simulink model "FC_Test"  (R2023b)
settings: Solver=FixedStepAuto  StartTime=0.0  StopTime=inf  RelTol=1e-3  EnableMultiTasking=on
PreLoadFcn:
  | setupEnv()
undefined symbols (not defined in the file or in its folder): bits, sensors
libraries: stm32blockslib x31, simulink x7, stm32f4xxblockslib x2
settings Model: STM32="{\"DigitalPortRead\":{\"ID\":\"FC_Test:2\"},\"DigitalPortWrite\":{\"ID\":\"FC_Test:4\"},\"I2CControllerRead\":[{\"ID\":\"FC_Test:28\"},{\"ID\":\"FC_Test:50\"},{\"ID\":\"FC_Test:52\"},{\"ID\":\"FC_Test:53\"},{\"ID\":\"FC_Test:68\"},{\"ID\":\"FC_Test:96\"},{\"ID\":\"FC_Test:191\"},{\"ID\":\"FC_Test:128\"},{\"ID\":\"FC_Test:121\"},{\"ID\":\"FC_Test:169\"},{\"ID\":\"FC_Test:249\"},{\"ID\":\"FC_Test:250\"},{\"ID\":\"FC_Test:237\"}],\"I2CControllerWrite\":[{\"ID\":\"FC_Test:86\"},{\"ID\":\"FC_Test:109\"},{\"ID\":\"FC_Test:94\"},{\"ID\":\"FC_Test:208\"},{\"ID\":\"FC_Test:192\"},{\"ID\":\"FC_Test:202\"},{\"ID\":\"FC_Test:140\"},{\"ID\":\"FC_Test:141\"},{\"ID\":\"FC_Test:142\"},{\"ID\":\"FC_Test:122\"},{\"ID\":\"FC_Test:170\"},{\"ID\":\"FC_Test:239\"},{\"ID\":\"FC_Test:242\"},{\"ID\":\"FC_Test:243\"},{\"ID\":\"FC_Test:246\"},{\"ID\":\"FC_Test:247\"},{\"ID\":\"FC_Test:255\"},{\"ID\":\"FC_Test:252\"}]}"  SimulationMode=external  Creator=Blind  LastModifiedBy=Blind
settings SolverCC: PositivePriorityOrder=on
settings OptimizationCC: EnhancedBackFolding=on  PassReuseOutputArgsAs=Individual arguments  ZeroExternalMemoryAtStartup=off  ZeroInternalMemoryAtStartup=off  MaxStackSize=64  OptimizeBlockOrder=speed  DifferentSizesBufferReuse=on  OptimizationCustomize=off  EfficientTunableParamExpr=on
settings DebuggingCC: ParameterTunabilityLossMsg=error
settings HardwareCC: ProdBitPerPointer=32  ProdBitPerSizeT=32  ProdBitPerPtrDiffT=32  ProdLargestAtomicInteger=Long  ProdLargestAtomicFloat=Double  ProdWordSize=32  ProdLongLongMode=on  ProdHWDeviceType=ARM Compatible->ARM Cortex
settings SFSimCC: MATLABDynamicMemAlloc=off
settings RTWCC: Description=Embedded Coder  SystemTargetFile=ert.tlc  HardwareBoard=STM32H7xx Based (Single-core)  TLCOptions="-aInlineSetEventsForThisBaseRateFcn=TLC_FALSE -aSuppressMultiTaskScheduler=TLC_FALSE   -aRateBasedStepFcn=1"  TemplateMakefile=ert_default_tmf  Toolchain=GNU Tools for ARM Embedded Processors
settings CodeAppCC: ForceParamTrailComments=on  IgnoreCustomStorageClasses=off  OperatorAnnotations=on  SimulinkDataObjDesc=on  SFDataObjDesc=on  InsertBlockDesc=on
settings ERTTargetCC: CodeReplacementLibrary=ARM Cortex-M  SupportContinuousTime=on  ExtModeTransport=3  ExtModeStaticAlloc=on  ExtModeStaticAllocSize=4096  ExtModeMexFile=ext_xcp  ExtModeIntrfLevel=Level2 - Open

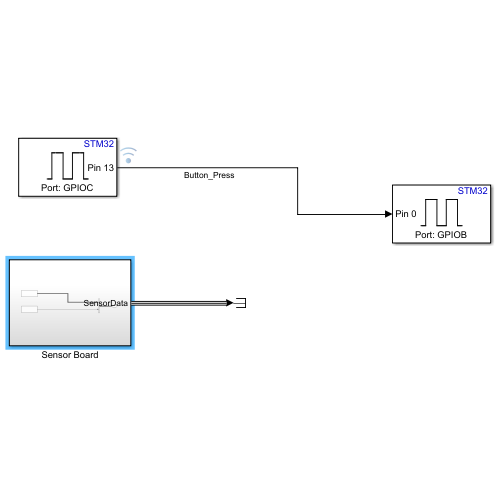
[thumbnail: Simulink's stored preview of the top-level diagram]
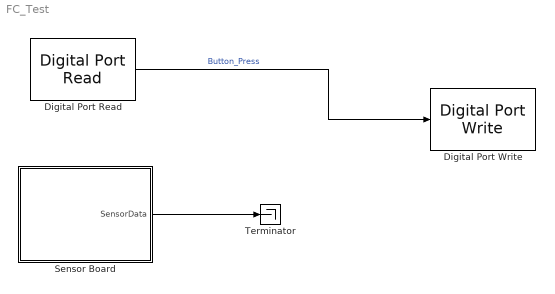
== system FC_Test ==
  Digital Port Read : stm32f4xxblockslib/Digital Port Read  PortName=GPIOC  PinNumber=13  ReadOperation=on  IOAsArray=off  SampleTime=-1  EnableSimPort=off  hoistedMaskSrc=ECSoC/ECSimCodegen/Digital Port Read
      settings: LibrarySourceBlock=stm32h7xxblockslib/Digital Port Read
  Digital Port Write : stm32f4xxblockslib/Digital Port Write  PortName=GPIOB  PinNumber=0  ReadOperation=off  IOAsArray=off  EnableSimPort=off  hoistedMaskSrc=ECSoC/ECSimCodegen/Digital Port Write
      settings: LibrarySourceBlock=stm32h7xxblockslib/Digital Port Write
  Sensor Board : Subsystem
  Terminator : Terminator
  wires:
  Digital Port Read/1 -> Digital Port Write/1  "Button_Press"
  Sensor Board/1(SensorData) -> Terminator/1

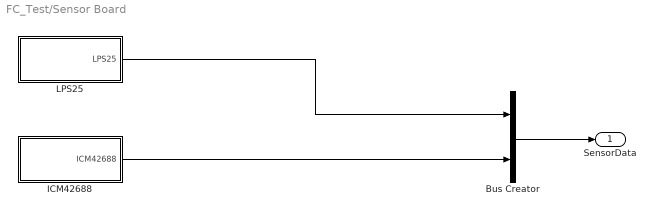
== system FC_Test/Sensor Board ==
  Bus Creator : BusCreator  Inputs=2
  ICM42688 : Subsystem
  LPS25 : Subsystem
  SensorData : Outport
  wires:
  LPS25/1(LPS25) -> Bus Creator/1
  Bus Creator/1 -> SensorData/1
  ICM42688/1(ICM42688) -> Bus Creator/2

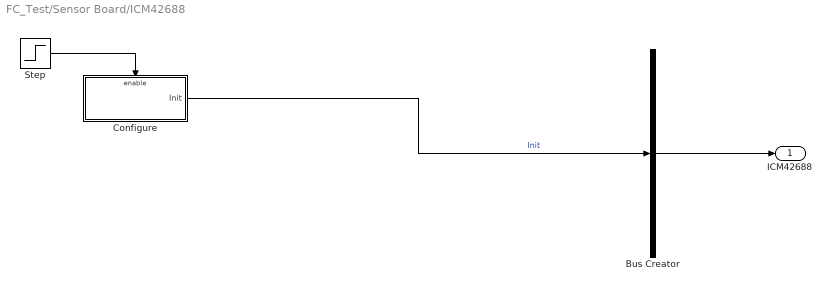
== system FC_Test/Sensor Board/ICM42688 ==
  Bus Creator : BusCreator  Inputs=1
  Configure : Subsystem
  Step : Step  Time=0  SampleTime=0
  ICM42688 : Outport
  wires:
  Configure/1(Init) -> Bus Creator/1  "Init"
  Step/1 -> Configure/Enable
  Bus Creator/1 -> ICM42688/1

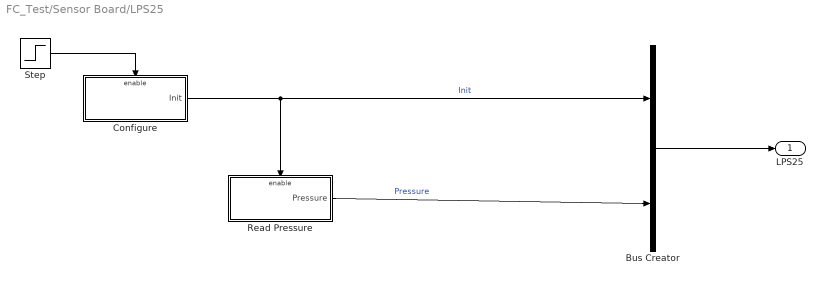
== system FC_Test/Sensor Board/LPS25 ==
  Bus Creator : BusCreator  Inputs=2
  Configure : Subsystem
  Read Pressure : Subsystem
  Step : Step  Time=0  SampleTime=0
  LPS25 : Outport
  wires:
  Step/1 -> Configure/Enable
  Read Pressure/1(Pressure) -> Bus Creator/2  "Pressure"
  Bus Creator/1 -> LPS25/1
  Configure/1(Init) -> Bus Creator/1, Read Pressure/Enable  "Init"

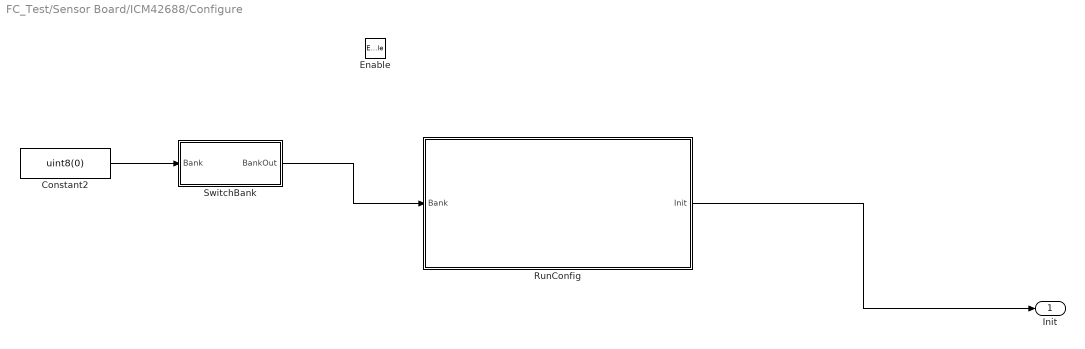
== system FC_Test/Sensor Board/ICM42688/Configure ==
  Enable : EnablePort
  Constant2 : Constant  Value=uint8(0)
  RunConfig : Subsystem
  SwitchBank : Subsystem
  Init : Outport
  wires:
  Constant2/1 -> SwitchBank/1(Bank)
  RunConfig/1(Init) -> Init/1
  SwitchBank/1(BankOut) -> RunConfig/1(Bank)

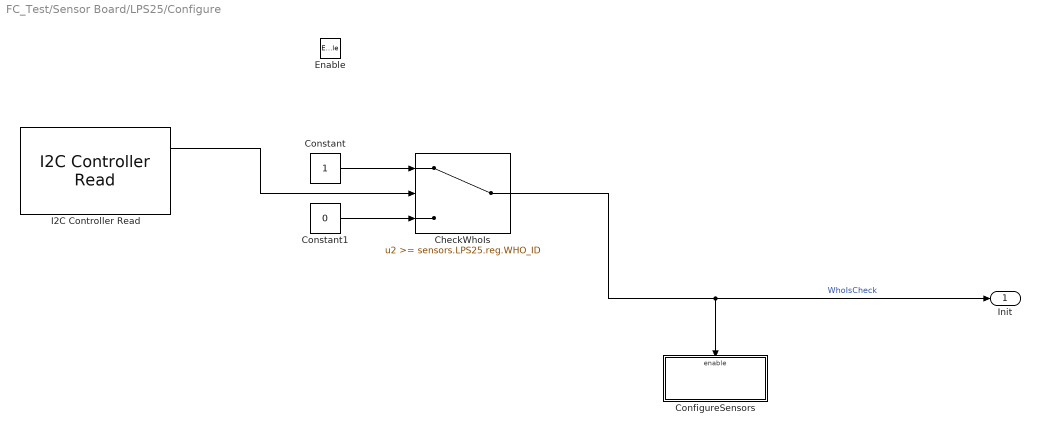
== system FC_Test/Sensor Board/LPS25/Configure ==
  Enable : EnablePort
  CheckWhoIs : Switch  Threshold=sensors.LPS25.reg.WHO_ID  SaturateOnIntegerOverflow=off  InputSameDT=off
  ConfigureSensors : Subsystem
  Constant : Constant
  Constant1 : Constant  Value=0
  I2C Controller Read : stm32blockslib/I2C Controller Read  I2CModule=I2C1  Mode=Controller  AddressingMode=7-bits  PeripheralByteOrder=BigEndian  OwnPeripheralAddress=uint8(170)  PeripheralAddressVia=Dialog  PeripheralAddress=sensors.LPS25.reg.ADDR  RegisterAddressMode=on  RegisterAddressVia=Dialog  RegisterAddress=sensors.LPS25.reg.WHOAMI  RepeatedStart=off  NoAck=off  OutputStatus=on  BlockMode=Receive  DataType=uint8  DataLength=1  Timeout=0.001  SampleTime=-1
      settings: LibrarySourceBlock=stm32h7xxblockslib/I2C Controller Read
  Init : Outport
  wires:
  I2C Controller Read/1 -> CheckWhoIs/2
  Constant/1 -> CheckWhoIs/1
  Constant1/1 -> CheckWhoIs/3
  CheckWhoIs/1 -> ConfigureSensors/Enable, Init/1  "WhoIsCheck"

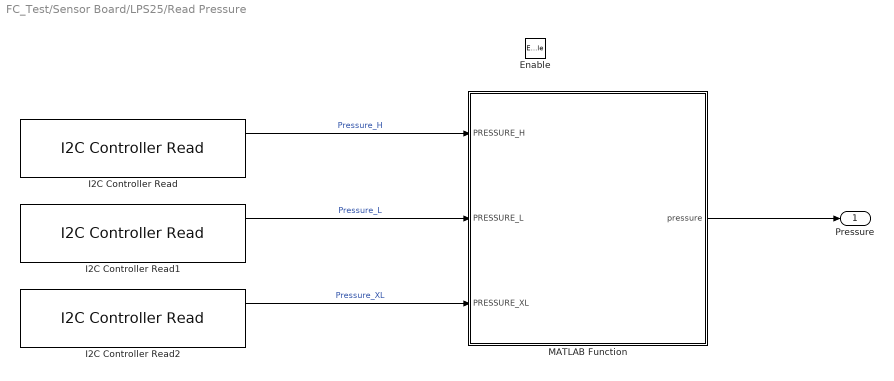
== system FC_Test/Sensor Board/LPS25/Read Pressure ==
  Enable : EnablePort
  I2C Controller Read : stm32blockslib/I2C Controller Read  I2CModule=I2C1  Mode=Controller  AddressingMode=7-bits  PeripheralByteOrder=BigEndian  OwnPeripheralAddress=uint8(170)  PeripheralAddressVia=Dialog  PeripheralAddress=sensors.LPS25.reg.ADDR  RegisterAddressMode=on  RegisterAddressVia=Dialog  RegisterAddress=sensors.LPS25.reg.PRESSURE_H_REG  RepeatedStart=off  NoAck=off  OutputStatus=on  BlockMode=Receive  DataType=uint8  DataLength=1  Timeout=0.001  SampleTime=-1
      settings: LibrarySourceBlock=stm32h7xxblockslib/I2C Controller Read
  I2C Controller Read1 : stm32blockslib/I2C Controller Read  I2CModule=I2C1  Mode=Controller  AddressingMode=7-bits  PeripheralByteOrder=BigEndian  OwnPeripheralAddress=uint8(170)  PeripheralAddressVia=Dialog  PeripheralAddress=sensors.LPS25.reg.ADDR  RegisterAddressMode=on  RegisterAddressVia=Dialog  RegisterAddress=sensors.LPS25.reg.PRESSURE_L_REG  RepeatedStart=off  NoAck=off  OutputStatus=on  BlockMode=Receive  DataType=uint8  DataLength=1  Timeout=0.001  SampleTime=-1
      settings: LibrarySourceBlock=stm32h7xxblockslib/I2C Controller Read
  I2C Controller Read2 : stm32blockslib/I2C Controller Read  I2CModule=I2C1  Mode=Controller  AddressingMode=7-bits  PeripheralByteOrder=BigEndian  OwnPeripheralAddress=uint8(170)  PeripheralAddressVia=Dialog  PeripheralAddress=sensors.LPS25.reg.ADDR  RegisterAddressMode=on  RegisterAddressVia=Dialog  RegisterAddress=sensors.LPS25.reg.PRESSURE_OUT_XL  RepeatedStart=off  NoAck=off  OutputStatus=on  BlockMode=Receive  DataType=uint8  DataLength=1  Timeout=0.001  SampleTime=-1
      settings: LibrarySourceBlock=stm32h7xxblockslib/I2C Controller Read
  MATLAB Function : MATLAB Function  TreatAsAtomicUnit=on
  Pressure : Outport
  wires:
  I2C Controller Read/1 -> MATLAB Function/1(PRESSURE_H)  "Pressure_H"
  I2C Controller Read1/1 -> MATLAB Function/2(PRESSURE_L)  "Pressure_L"
  I2C Controller Read2/1 -> MATLAB Function/3(PRESSURE_XL)  "Pressure_XL"
  MATLAB Function/1(pressure) -> Pressure/1

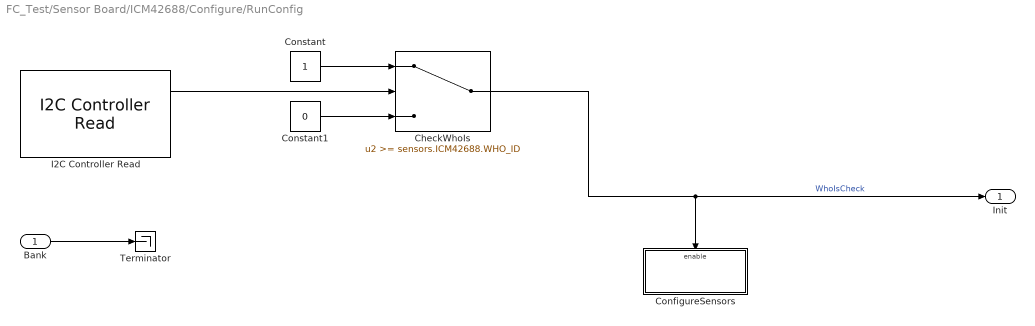
== system FC_Test/Sensor Board/ICM42688/Configure/RunConfig ==
  Bank : Inport
  CheckWhoIs : Switch  Threshold=sensors.ICM42688.WHO_ID  SaturateOnIntegerOverflow=off  InputSameDT=off
  ConfigureSensors : Subsystem
  Constant : Constant
  Constant1 : Constant  Value=0
  I2C Controller Read : stm32blockslib/I2C Controller Read  I2CModule=I2C1  Mode=Controller  AddressingMode=7-bits  PeripheralByteOrder=BigEndian  OwnPeripheralAddress=uint8(170)  PeripheralAddressVia=Dialog  PeripheralAddress=sensors.ICM42688.reg.ADDR  RegisterAddressMode=on  RegisterAddressVia=Dialog  RegisterAddress=sensors.ICM42688.reg.BANK0.WHO_AM_I  RepeatedStart=off  NoAck=off  OutputStatus=on  BlockMode=Receive  DataType=uint8  DataLength=1  Timeout=0.001  SampleTime=-1
      settings: LibrarySourceBlock=stm32h7xxblockslib/I2C Controller Read
  Terminator : Terminator
  Init : Outport
  wires:
  I2C Controller Read/1 -> CheckWhoIs/2
  CheckWhoIs/1 -> Init/1, ConfigureSensors/Enable  "WhoIsCheck"
  Constant/1 -> CheckWhoIs/1
  Constant1/1 -> CheckWhoIs/3
  Bank/1 -> Terminator/1

== system FC_Test/Sensor Board/ICM42688/Configure/SwitchBank ==
  Bank : Inport
  I2C Controller Read : stm32blockslib/I2C Controller Read  I2CModule=I2C1  Mode=Controller  AddressingMode=7-bits  PeripheralByteOrder=BigEndian  OwnPeripheralAddress=uint8(170)  PeripheralAddressVia=Dialog  PeripheralAddress=sensors.ICM42688.reg.ADDR  RegisterAddressMode=on  RegisterAddressVia=Dialog  RegisterAddress=sensors.ICM42688.reg.REG_BANK_SEL  RepeatedStart=off  NoAck=off  OutputStatus=on  BlockMode=Receive  DataType=uint8  DataLength=1  Timeout=0.001  SampleTime=-1
      settings: LibrarySourceBlock=stm32h7xxblockslib/I2C Controller Read
  I2C Controller Write : stm32blockslib/I2C Controller Write  I2CModule=I2C1  Mode=Controller  AddressingMode=7-bits  PeripheralByteOrder=BigEndian  OwnPeripheralAddress=uint8(170)  PeripheralAddressVia=Dialog  PeripheralAddress=sensors.ICM42688.reg.ADDR  RegisterAddressMode=on  RegisterAddressVia=Dialog  RegisterAddress=sensors.ICM42688.reg.REG_BANK_SEL  RepeatedStart=off  NoAck=off  OutputStatus=on  BlockMode=Transmit  DataType=uint8  DataLength=1  Timeout=0.001  SampleTime=-1
      settings: LibrarySourceBlock=stm32h7xxblockslib/I2C Controller Write
  BankOut : Outport
  wires:
  Bank/1 -> I2C Controller Write/1
  I2C Controller Read/1 -> BankOut/1

== system FC_Test/Sensor Board/LPS25/Configure/ConfigureSensors ==
  Enable : EnablePort
  Constant : Constant  Value=sensors.LPS25.config.ODR.Hz25
  I2C Controller Write : stm32blockslib/I2C Controller Write  I2CModule=I2C1  Mode=Controller  AddressingMode=7-bits  PeripheralByteOrder=BigEndian  OwnPeripheralAddress=uint8(170)  PeripheralAddressVia=Dialog  PeripheralAddress=sensors.LPS25.reg.ADDR  RegisterAddressMode=on  RegisterAddressVia=Dialog  RegisterAddress=sensors.LPS25.reg.CTRL1  RepeatedStart=off  NoAck=off  OutputStatus=on  BlockMode=Transmit  DataType=uint8  DataLength=1  Timeout=0.001  SampleTime=-1
      settings: LibrarySourceBlock=stm32h7xxblockslib/I2C Controller Write
  wires:
  Constant/1 -> I2C Controller Write/1

== system FC_Test/Sensor Board/ICM42688/Configure/RunConfig/ConfigureSensors ==
  Enable : EnablePort
  EnableSensor : Subsystem
  SetFilters : Subsystem
  SetODR : Subsystem

== system FC_Test/Sensor Board/ICM42688/Configure/RunConfig/ConfigureSensors/EnableSensor ==
  Constant : Constant  Value=sensors.ICM42688.config.SENSOR_ENABLE
  I2C Controller Write : stm32blockslib/I2C Controller Write  I2CModule=I2C1  Mode=Controller  AddressingMode=7-bits  PeripheralByteOrder=BigEndian  OwnPeripheralAddress=uint8(170)  PeripheralAddressVia=Dialog  PeripheralAddress=sensors.ICM42688.reg.ADDR  RegisterAddressMode=on  RegisterAddressVia=Dialog  RegisterAddress=sensors.ICM42688.reg.BANK0.PWR_MGMT0  RepeatedStart=off  NoAck=off  OutputStatus=on  BlockMode=Transmit  DataType=uint8  DataLength=1  Timeout=0.001  SampleTime=-1
      settings: LibrarySourceBlock=stm32h7xxblockslib/I2C Controller Write
  Status : Outport
  wires:
  Constant/1 -> I2C Controller Write/1
  I2C Controller Write/1 -> Status/1

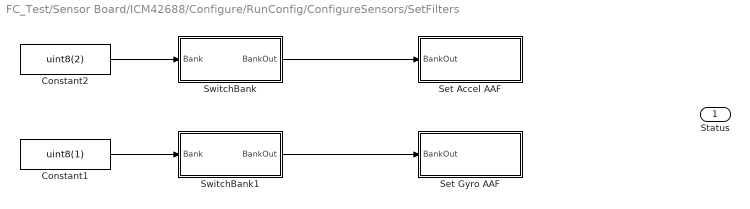
== system FC_Test/Sensor Board/ICM42688/Configure/RunConfig/ConfigureSensors/SetFilters ==
  Constant1 : Constant  Value=uint8(1)
  Constant2 : Constant  Value=uint8(2)
  Set Accel AAF : Subsystem
  Set Gyro AAF : Subsystem
  SwitchBank : Subsystem
  SwitchBank1 : Subsystem
  Status : Outport
  wires:
  Constant2/1 -> SwitchBank/1(Bank)
  SwitchBank/1(BankOut) -> Set Accel AAF/1(BankOut)
  Constant1/1 -> SwitchBank1/1(Bank)
  SwitchBank1/1(BankOut) -> Set Gyro AAF/1(BankOut)

== system FC_Test/Sensor Board/ICM42688/Configure/RunConfig/ConfigureSensors/SetODR ==
  Constant1 : Constant  Value=uint8(0)
  ODR : Subsystem
  SwitchBank1 : Subsystem
  Status : Outport
  wires:
  Constant1/1 -> SwitchBank1/1(Bank)
  SwitchBank1/1(BankOut) -> ODR/1(BankOut)
  ODR/1(Out1) -> Status/1

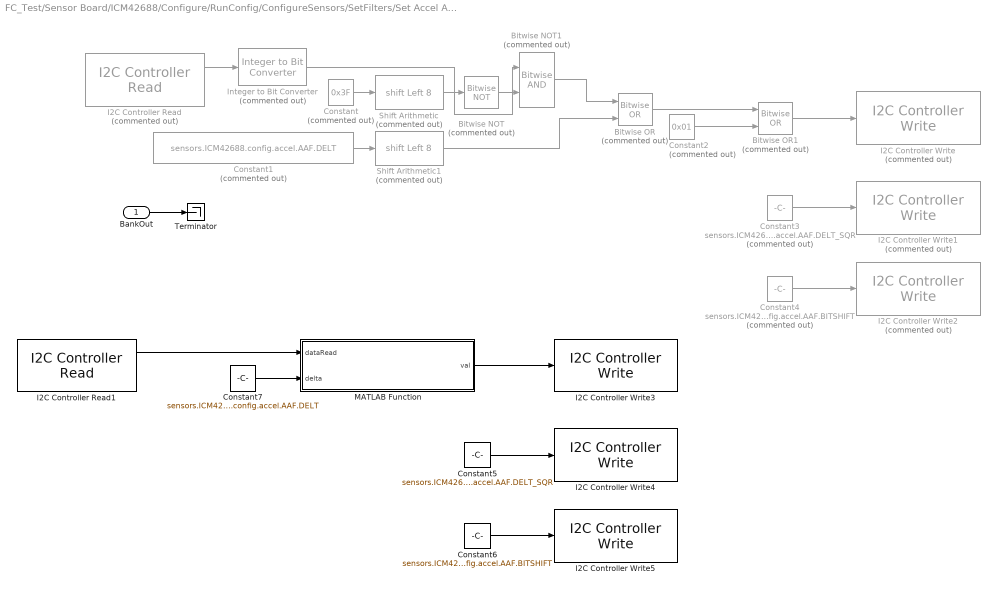
== system FC_Test/Sensor Board/ICM42688/Configure/RunConfig/ConfigureSensors/SetFilters/Set Accel AAF ==
  BankOut : Inport
  Bitwise NOT : simulink/Logic and Bit Operations/Bitwise Operator  Commented=on  logicop=NOT  UseBitMask=off  BitMask=bin2dec('11011001')  BitMaskRealWorld=Stored Integer
      settings: LibrarySourceBlock=|
      | simulink/Quick Insert/Logic and Bit
      | Operations/Bitwise NOT
  Bitwise NOT1 : simulink/Logic and Bit Operations/Bitwise Operator  Commented=on  logicop=AND  UseBitMask=off  NumInputPorts=2  BitMask=bin2dec('11011001')  BitMaskRealWorld=Stored Integer
      settings: LibrarySourceBlock=|
      | simulink/Quick Insert/Logic and Bit
      | Operations/Bitwise NOT
  Bitwise OR : simulink/Logic and Bit Operations/Bitwise Operator  Commented=on  logicop=OR  UseBitMask=off  NumInputPorts=2  BitMask=bin2dec('11011001')  BitMaskRealWorld=Stored Integer
      settings: LibrarySourceBlock=|
      | simulink/Quick Insert/Logic and Bit
      | Operations/Bitwise OR
  Bitwise OR1 : simulink/Logic and Bit Operations/Bitwise Operator  Commented=on  logicop=OR  UseBitMask=off  NumInputPorts=2  BitMask=bin2dec('11011001')  BitMaskRealWorld=Stored Integer
      settings: LibrarySourceBlock=|
      | simulink/Quick Insert/Logic and Bit
      | Operations/Bitwise OR
  Constant : Constant  Commented=on  Value=0x3F
  Constant1 : Constant  Commented=on  Value=sensors.ICM42688.config.accel.AAF.DELT
  Constant2 : Constant  Commented=on  Value=0x01
  Constant3 : Constant  Commented=on  Value=sensors.ICM42688.config.accel.AAF.DELT_SQR
  Constant4 : Constant  Commented=on  Value=sensors.ICM42688.config.accel.AAF.BITSHIFT
  Constant5 : Constant  Value=sensors.ICM42688.config.accel.AAF.DELT_SQR
  Constant6 : Constant  Value=sensors.ICM42688.config.accel.AAF.BITSHIFT
  Constant7 : Constant  Value=sensors.ICM42688.config.accel.AAF.DELT
  I2C Controller Read : stm32blockslib/I2C Controller Read  Commented=on  I2CModule=I2C1  Mode=Controller  AddressingMode=7-bits  PeripheralByteOrder=BigEndian  OwnPeripheralAddress=uint8(170)  PeripheralAddressVia=Dialog  PeripheralAddress=sensors.ICM42688.reg.ADDR  RegisterAddressMode=on  RegisterAddressVia=Dialog  RegisterAddress=sensors.ICM42688.reg.BANK2.ACCEL_CONFIG_STATIC2  RepeatedStart=off  NoAck=off  OutputStatus=on  BlockMode=Receive  DataType=uint8  DataLength=1  Timeout=0.001  SampleTime=-1
      settings: LibrarySourceBlock=stm32h7xxblockslib/I2C Controller Read
  I2C Controller Read1 : stm32blockslib/I2C Controller Read  I2CModule=I2C1  Mode=Controller  AddressingMode=7-bits  PeripheralByteOrder=BigEndian  OwnPeripheralAddress=uint8(170)  PeripheralAddressVia=Dialog  PeripheralAddress=sensors.ICM42688.reg.ADDR  RegisterAddressMode=on  RegisterAddressVia=Dialog  RegisterAddress=sensors.ICM42688.reg.BANK2.ACCEL_CONFIG_STATIC2  RepeatedStart=off  NoAck=off  OutputStatus=on  BlockMode=Receive  DataType=uint8  DataLength=1  Timeout=0.001  SampleTime=-1
      settings: LibrarySourceBlock=stm32h7xxblockslib/I2C Controller Read
  I2C Controller Write : stm32blockslib/I2C Controller Write  Commented=on  I2CModule=I2C1  Mode=Controller  AddressingMode=7-bits  PeripheralByteOrder=BigEndian  OwnPeripheralAddress=uint8(170)  PeripheralAddressVia=Dialog  PeripheralAddress=sensors.ICM42688.reg.ADDR  RegisterAddressMode=on  RegisterAddressVia=Dialog  RegisterAddress=sensors.ICM42688.reg.BANK2.ACCEL_CONFIG_STATIC2  RepeatedStart=off  NoAck=off  OutputStatus=on  BlockMode=Transmit  DataType=uint8  DataLength=1  Timeout=0.001  SampleTime=-1
      settings: LibrarySourceBlock=stm32h7xxblockslib/I2C Controller Write
  I2C Controller Write1 : stm32blockslib/I2C Controller Write  Commented=on  I2CModule=I2C1  Mode=Controller  AddressingMode=7-bits  PeripheralByteOrder=BigEndian  OwnPeripheralAddress=uint8(170)  PeripheralAddressVia=Dialog  PeripheralAddress=sensors.ICM42688.reg.ADDR  RegisterAddressMode=on  RegisterAddressVia=Dialog  RegisterAddress=sensors.ICM42688.reg.BANK2.ACCEL_CONFIG_STATIC3  RepeatedStart=off  NoAck=off  OutputStatus=on  BlockMode=Transmit  DataType=uint8  DataLength=1  Timeout=0.001  SampleTime=-1
      settings: LibrarySourceBlock=stm32h7xxblockslib/I2C Controller Write
  I2C Controller Write2 : stm32blockslib/I2C Controller Write  Commented=on  I2CModule=I2C1  Mode=Controller  AddressingMode=7-bits  PeripheralByteOrder=BigEndian  OwnPeripheralAddress=uint8(170)  PeripheralAddressVia=Dialog  PeripheralAddress=sensors.ICM42688.reg.ADDR  RegisterAddressMode=on  RegisterAddressVia=Dialog  RegisterAddress=sensors.ICM42688.reg.BANK2.ACCEL_CONFIG_STATIC4  RepeatedStart=off  NoAck=off  OutputStatus=on  BlockMode=Transmit  DataType=uint8  DataLength=1  Timeout=0.001  SampleTime=-1
      settings: LibrarySourceBlock=stm32h7xxblockslib/I2C Controller Write
  I2C Controller Write3 : stm32blockslib/I2C Controller Write  I2CModule=I2C1  Mode=Controller  AddressingMode=7-bits  PeripheralByteOrder=BigEndian  OwnPeripheralAddress=uint8(170)  PeripheralAddressVia=Dialog  PeripheralAddress=sensors.ICM42688.reg.ADDR  RegisterAddressMode=on  RegisterAddressVia=Dialog  RegisterAddress=sensors.ICM42688.reg.BANK2.ACCEL_CONFIG_STATIC2  RepeatedStart=off  NoAck=off  OutputStatus=on  BlockMode=Transmit  DataType=uint8  DataLength=1  Timeout=0.001  SampleTime=-1
      settings: LibrarySourceBlock=stm32h7xxblockslib/I2C Controller Write
  I2C Controller Write4 : stm32blockslib/I2C Controller Write  I2CModule=I2C1  Mode=Controller  AddressingMode=7-bits  PeripheralByteOrder=BigEndian  OwnPeripheralAddress=uint8(170)  PeripheralAddressVia=Dialog  PeripheralAddress=sensors.ICM42688.reg.ADDR  RegisterAddressMode=on  RegisterAddressVia=Dialog  RegisterAddress=sensors.ICM42688.reg.BANK2.ACCEL_CONFIG_STATIC3  RepeatedStart=off  NoAck=off  OutputStatus=on  BlockMode=Transmit  DataType=uint8  DataLength=1  Timeout=0.001  SampleTime=-1
      settings: LibrarySourceBlock=stm32h7xxblockslib/I2C Controller Write
  I2C Controller Write5 : stm32blockslib/I2C Controller Write  I2CModule=I2C1  Mode=Controller  AddressingMode=7-bits  PeripheralByteOrder=BigEndian  OwnPeripheralAddress=uint8(170)  PeripheralAddressVia=Dialog  PeripheralAddress=sensors.ICM42688.reg.ADDR  RegisterAddressMode=on  RegisterAddressVia=Dialog  RegisterAddress=sensors.ICM42688.reg.BANK2.ACCEL_CONFIG_STATIC4  RepeatedStart=off  NoAck=off  OutputStatus=on  BlockMode=Transmit  DataType=uint8  DataLength=1  Timeout=0.001  SampleTime=-1
      settings: LibrarySourceBlock=stm32h7xxblockslib/I2C Controller Write
  Integer to Bit Converter : simulink/Logic and Bit Operations/Integer to Bit Converter  Commented=on  nbits=3  signedInputValues=Unsigned  bitOrder=MSB first  outDtype=Inherit via internal rule
  MATLAB Function : MATLAB Function  TreatAsAtomicUnit=on
  Shift Arithmetic : ArithShift  Commented=on  BitShiftNumber=8  BinPtShiftNumber=1  BitShiftDirection=Left
  Shift Arithmetic1 : ArithShift  Commented=on  BitShiftNumber=8  BinPtShiftNumber=1  BitShiftDirection=Left
  Terminator : Terminator
  wires:
  BankOut/1 -> Terminator/1
  Constant/1 -> Shift Arithmetic/1
  Shift Arithmetic/1 -> Bitwise NOT/1
  I2C Controller Read/1 -> Integer to Bit Converter/1
  Constant1/1 -> Shift Arithmetic1/1
  Shift Arithmetic1/1 -> Bitwise OR/2
  Bitwise OR/1 -> Bitwise OR1/1
  Constant2/1 -> Bitwise OR1/2
  Bitwise OR1/1 -> I2C Controller Write/1
  Constant3/1 -> I2C Controller Write1/1
  Constant4/1 -> I2C Controller Write2/1
  Bitwise NOT1/1 -> Bitwise OR/1
  Bitwise NOT/1 -> Bitwise NOT1/2
  Integer to Bit Converter/1 -> Bitwise NOT1/1
  I2C Controller Read1/1 -> MATLAB Function/1(dataRead)
  MATLAB Function/1(val) -> I2C Controller Write3/1
  Constant5/1 -> I2C Controller Write4/1
  Constant6/1 -> I2C Controller Write5/1
  Constant7/1 -> MATLAB Function/2(delta)

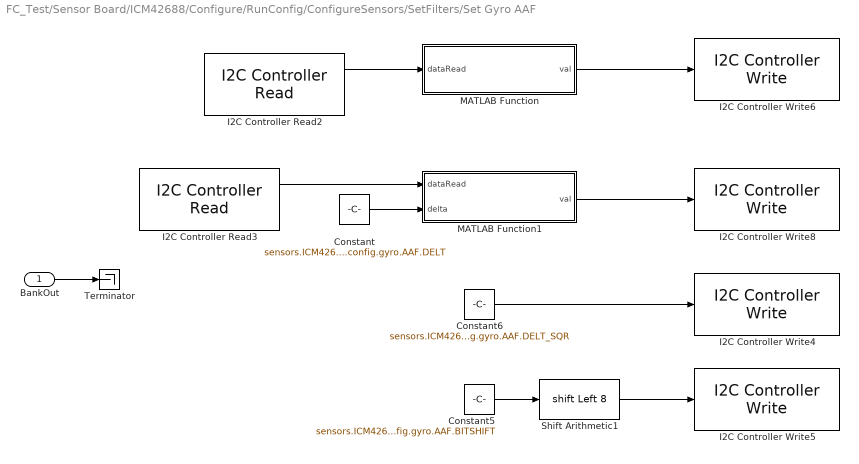
== system FC_Test/Sensor Board/ICM42688/Configure/RunConfig/ConfigureSensors/SetFilters/Set Gyro AAF ==
  BankOut : Inport
  Constant : Constant  Value=sensors.ICM42688.config.gyro.AAF.DELT
  Constant5 : Constant  Value=sensors.ICM42688.config.gyro.AAF.BITSHIFT
  Constant6 : Constant  Value=sensors.ICM42688.config.gyro.AAF.DELT_SQR
  I2C Controller Read2 : stm32blockslib/I2C Controller Read  I2CModule=I2C1  Mode=Controller  AddressingMode=7-bits  PeripheralByteOrder=BigEndian  OwnPeripheralAddress=uint8(170)  PeripheralAddressVia=Dialog  PeripheralAddress=sensors.ICM42688.reg.ADDR  RegisterAddressMode=on  RegisterAddressVia=Dialog  RegisterAddress=sensors.ICM42688.reg.BANK1.GYRO_CONFIG_STATIC2  RepeatedStart=off  NoAck=off  OutputStatus=on  BlockMode=Receive  DataType=uint8  DataLength=1  Timeout=0.001  SampleTime=-1
      settings: LibrarySourceBlock=stm32h7xxblockslib/I2C Controller Read
  I2C Controller Read3 : stm32blockslib/I2C Controller Read  I2CModule=I2C1  Mode=Controller  AddressingMode=7-bits  PeripheralByteOrder=BigEndian  OwnPeripheralAddress=uint8(170)  PeripheralAddressVia=Dialog  PeripheralAddress=sensors.ICM42688.reg.ADDR  RegisterAddressMode=on  RegisterAddressVia=Dialog  RegisterAddress=sensors.ICM42688.reg.BANK1.GYRO_CONFIG_STATIC3  RepeatedStart=off  NoAck=off  OutputStatus=on  BlockMode=Receive  DataType=uint8  DataLength=1  Timeout=0.001  SampleTime=-1
      settings: LibrarySourceBlock=stm32h7xxblockslib/I2C Controller Read
  I2C Controller Write4 : stm32blockslib/I2C Controller Write  I2CModule=I2C1  Mode=Controller  AddressingMode=7-bits  PeripheralByteOrder=BigEndian  OwnPeripheralAddress=uint8(170)  PeripheralAddressVia=Dialog  PeripheralAddress=sensors.ICM42688.reg.ADDR  RegisterAddressMode=on  RegisterAddressVia=Dialog  RegisterAddress=sensors.ICM42688.reg.BANK1.GYRO_CONFIG_STATIC4  RepeatedStart=off  NoAck=off  OutputStatus=on  BlockMode=Transmit  DataType=uint8  DataLength=1  Timeout=0.001  SampleTime=-1
      settings: LibrarySourceBlock=stm32h7xxblockslib/I2C Controller Write
  I2C Controller Write5 : stm32blockslib/I2C Controller Write  I2CModule=I2C1  Mode=Controller  AddressingMode=7-bits  PeripheralByteOrder=BigEndian  OwnPeripheralAddress=uint8(170)  PeripheralAddressVia=Dialog  PeripheralAddress=sensors.ICM42688.reg.ADDR  RegisterAddressMode=on  RegisterAddressVia=Dialog  RegisterAddress=sensors.ICM42688.reg.BANK1.GYRO_CONFIG_STATIC5  RepeatedStart=off  NoAck=off  OutputStatus=on  BlockMode=Transmit  DataType=uint8  DataLength=1  Timeout=0.001  SampleTime=-1
      settings: LibrarySourceBlock=stm32h7xxblockslib/I2C Controller Write
  I2C Controller Write6 : stm32blockslib/I2C Controller Write  I2CModule=I2C1  Mode=Controller  AddressingMode=7-bits  PeripheralByteOrder=BigEndian  OwnPeripheralAddress=uint8(170)  PeripheralAddressVia=Dialog  PeripheralAddress=sensors.ICM42688.reg.ADDR  RegisterAddressMode=on  RegisterAddressVia=Dialog  RegisterAddress=sensors.ICM42688.reg.BANK1.GYRO_CONFIG_STATIC2  RepeatedStart=off  NoAck=off  OutputStatus=on  BlockMode=Transmit  DataType=uint8  DataLength=1  Timeout=0.001  SampleTime=-1
      settings: LibrarySourceBlock=stm32h7xxblockslib/I2C Controller Write
  I2C Controller Write8 : stm32blockslib/I2C Controller Write  I2CModule=I2C1  Mode=Controller  AddressingMode=7-bits  PeripheralByteOrder=BigEndian  OwnPeripheralAddress=uint8(170)  PeripheralAddressVia=Dialog  PeripheralAddress=sensors.ICM42688.reg.ADDR  RegisterAddressMode=on  RegisterAddressVia=Dialog  RegisterAddress=sensors.ICM42688.reg.BANK1.GYRO_CONFIG_STATIC3  RepeatedStart=off  NoAck=off  OutputStatus=on  BlockMode=Transmit  DataType=uint8  DataLength=1  Timeout=0.001  SampleTime=-1
      settings: LibrarySourceBlock=stm32h7xxblockslib/I2C Controller Write
  MATLAB Function : MATLAB Function  TreatAsAtomicUnit=on
  MATLAB Function1 : MATLAB Function  TreatAsAtomicUnit=on
  Shift Arithmetic1 : ArithShift  BitShiftNumber=8  BinPtShiftNumber=4  BitShiftDirection=Left
  Terminator : Terminator
  wires:
  BankOut/1 -> Terminator/1
  Constant6/1 -> I2C Controller Write4/1
  Constant5/1 -> Shift Arithmetic1/1
  Shift Arithmetic1/1 -> I2C Controller Write5/1
  I2C Controller Read2/1 -> MATLAB Function/1(dataRead)
  MATLAB Function/1(val) -> I2C Controller Write6/1
  I2C Controller Read3/1 -> MATLAB Function1/1(dataRead)
  MATLAB Function1/1(val) -> I2C Controller Write8/1
  Constant/1 -> MATLAB Function1/2(delta)

== system FC_Test/Sensor Board/ICM42688/Configure/RunConfig/ConfigureSensors/SetFilters/SwitchBank ==
  Bank : Inport
  I2C Controller Read : stm32blockslib/I2C Controller Read  I2CModule=I2C1  Mode=Controller  AddressingMode=7-bits  PeripheralByteOrder=BigEndian  OwnPeripheralAddress=uint8(170)  PeripheralAddressVia=Dialog  PeripheralAddress=sensors.ICM42688.reg.ADDR  RegisterAddressMode=on  RegisterAddressVia=Dialog  RegisterAddress=sensors.ICM42688.reg.REG_BANK_SEL  RepeatedStart=off  NoAck=off  OutputStatus=on  BlockMode=Receive  DataType=uint8  DataLength=1  Timeout=0.001  SampleTime=-1
      settings: LibrarySourceBlock=stm32h7xxblockslib/I2C Controller Read
  I2C Controller Write : stm32blockslib/I2C Controller Write  I2CModule=I2C1  Mode=Controller  AddressingMode=7-bits  PeripheralByteOrder=BigEndian  OwnPeripheralAddress=uint8(170)  PeripheralAddressVia=Dialog  PeripheralAddress=sensors.ICM42688.reg.ADDR  RegisterAddressMode=on  RegisterAddressVia=Dialog  RegisterAddress=sensors.ICM42688.reg.REG_BANK_SEL  RepeatedStart=off  NoAck=off  OutputStatus=on  BlockMode=Transmit  DataType=uint8  DataLength=1  Timeout=0.001  SampleTime=-1
      settings: LibrarySourceBlock=stm32h7xxblockslib/I2C Controller Write
  BankOut : Outport
  wires:
  Bank/1 -> I2C Controller Write/1
  I2C Controller Read/1 -> BankOut/1

== system FC_Test/Sensor Board/ICM42688/Configure/RunConfig/ConfigureSensors/SetFilters/SwitchBank1 ==
  Bank : Inport
  I2C Controller Read : stm32blockslib/I2C Controller Read  I2CModule=I2C1  Mode=Controller  AddressingMode=7-bits  PeripheralByteOrder=BigEndian  OwnPeripheralAddress=uint8(170)  PeripheralAddressVia=Dialog  PeripheralAddress=sensors.ICM42688.reg.ADDR  RegisterAddressMode=on  RegisterAddressVia=Dialog  RegisterAddress=sensors.ICM42688.reg.REG_BANK_SEL  RepeatedStart=off  NoAck=off  OutputStatus=on  BlockMode=Receive  DataType=uint8  DataLength=1  Timeout=0.001  SampleTime=-1
      settings: LibrarySourceBlock=stm32h7xxblockslib/I2C Controller Read
  I2C Controller Write : stm32blockslib/I2C Controller Write  I2CModule=I2C1  Mode=Controller  AddressingMode=7-bits  PeripheralByteOrder=BigEndian  OwnPeripheralAddress=uint8(170)  PeripheralAddressVia=Dialog  PeripheralAddress=sensors.ICM42688.reg.ADDR  RegisterAddressMode=on  RegisterAddressVia=Dialog  RegisterAddress=sensors.ICM42688.reg.REG_BANK_SEL  RepeatedStart=off  NoAck=off  OutputStatus=on  BlockMode=Transmit  DataType=uint8  DataLength=1  Timeout=0.001  SampleTime=-1
      settings: LibrarySourceBlock=stm32h7xxblockslib/I2C Controller Write
  BankOut : Outport
  wires:
  Bank/1 -> I2C Controller Write/1
  I2C Controller Read/1 -> BankOut/1

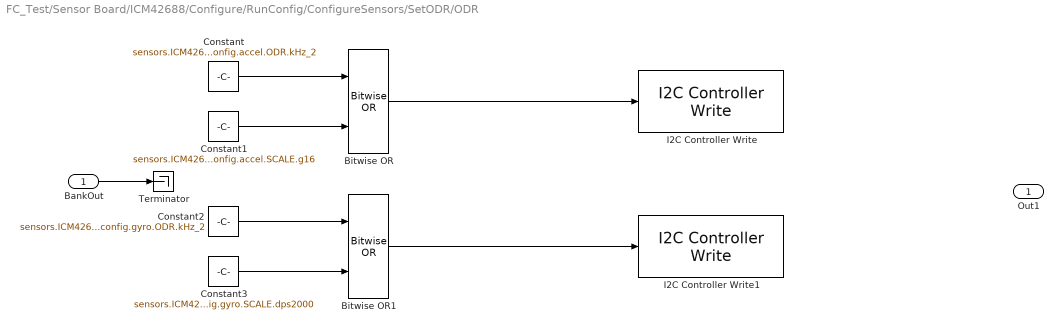
== system FC_Test/Sensor Board/ICM42688/Configure/RunConfig/ConfigureSensors/SetODR/ODR ==
  BankOut : Inport
  Bitwise OR : simulink/Logic and Bit Operations/Bitwise Operator  logicop=OR  UseBitMask=off  NumInputPorts=2  BitMask=bin2dec('11011001')  BitMaskRealWorld=Stored Integer
      settings: LibrarySourceBlock=|
      | simulink/Quick Insert/Logic and Bit
      | Operations/Bitwise OR
  Bitwise OR1 : simulink/Logic and Bit Operations/Bitwise Operator  logicop=OR  UseBitMask=off  NumInputPorts=2  BitMask=bin2dec('11011001')  BitMaskRealWorld=Stored Integer
      settings: LibrarySourceBlock=|
      | simulink/Quick Insert/Logic and Bit
      | Operations/Bitwise OR
  Constant : Constant  Value=sensors.ICM42688.config.accel.ODR.kHz_2
  Constant1 : Constant  Value=sensors.ICM42688.config.accel.SCALE.g16
  Constant2 : Constant  Value=sensors.ICM42688.config.gyro.ODR.kHz_2
  Constant3 : Constant  Value=sensors.ICM42688.config.gyro.SCALE.dps2000
  I2C Controller Write : stm32blockslib/I2C Controller Write  I2CModule=I2C1  Mode=Controller  AddressingMode=7-bits  PeripheralByteOrder=BigEndian  OwnPeripheralAddress=uint8(170)  PeripheralAddressVia=Dialog  PeripheralAddress=sensors.ICM42688.reg.ADDR  RegisterAddressMode=on  RegisterAddressVia=Dialog  RegisterAddress=sensors.ICM42688.reg.BANK0.ACCEL_CONFIG0  RepeatedStart=off  NoAck=off  OutputStatus=on  BlockMode=Transmit  DataType=uint8  DataLength=1  Timeout=0.001  SampleTime=-1
      settings: LibrarySourceBlock=stm32h7xxblockslib/I2C Controller Write
  I2C Controller Write1 : stm32blockslib/I2C Controller Write  I2CModule=I2C1  Mode=Controller  AddressingMode=7-bits  PeripheralByteOrder=BigEndian  OwnPeripheralAddress=uint8(170)  PeripheralAddressVia=Dialog  PeripheralAddress=sensors.ICM42688.reg.ADDR  RegisterAddressMode=on  RegisterAddressVia=Dialog  RegisterAddress=sensors.ICM42688.reg.BANK0.ACCEL_CONFIG0  RepeatedStart=off  NoAck=off  OutputStatus=on  BlockMode=Transmit  DataType=uint8  DataLength=1  Timeout=0.001  SampleTime=-1
      settings: LibrarySourceBlock=stm32h7xxblockslib/I2C Controller Write
  Terminator : Terminator
  Out1 : Outport
  wires:
  BankOut/1 -> Terminator/1
  Constant/1 -> Bitwise OR/1
  Constant1/1 -> Bitwise OR/2
  Bitwise OR/1 -> I2C Controller Write/1
  Constant2/1 -> Bitwise OR1/1
  Bitwise OR1/1 -> I2C Controller Write1/1
  Constant3/1 -> Bitwise OR1/2

== system FC_Test/Sensor Board/ICM42688/Configure/RunConfig/ConfigureSensors/SetODR/SwitchBank1 ==
  Bank : Inport
  I2C Controller Read : stm32blockslib/I2C Controller Read  I2CModule=I2C1  Mode=Controller  AddressingMode=7-bits  PeripheralByteOrder=BigEndian  OwnPeripheralAddress=uint8(170)  PeripheralAddressVia=Dialog  PeripheralAddress=sensors.ICM42688.reg.ADDR  RegisterAddressMode=on  RegisterAddressVia=Dialog  RegisterAddress=sensors.ICM42688.reg.REG_BANK_SEL  RepeatedStart=off  NoAck=off  OutputStatus=on  BlockMode=Receive  DataType=uint8  DataLength=1  Timeout=0.001  SampleTime=-1
      settings: LibrarySourceBlock=stm32h7xxblockslib/I2C Controller Read
  I2C Controller Write : stm32blockslib/I2C Controller Write  I2CModule=I2C1  Mode=Controller  AddressingMode=7-bits  PeripheralByteOrder=BigEndian  OwnPeripheralAddress=uint8(170)  PeripheralAddressVia=Dialog  PeripheralAddress=sensors.ICM42688.reg.ADDR  RegisterAddressMode=on  RegisterAddressVia=Dialog  RegisterAddress=sensors.ICM42688.reg.REG_BANK_SEL  RepeatedStart=off  NoAck=off  OutputStatus=on  BlockMode=Transmit  DataType=uint8  DataLength=1  Timeout=0.001  SampleTime=-1
      settings: LibrarySourceBlock=stm32h7xxblockslib/I2C Controller Write
  BankOut : Outport
  wires:
  Bank/1 -> I2C Controller Write/1
  I2C Controller Read/1 -> BankOut/1

== matlab function FC_Test/Sensor Board/LPS25/Read Pressure/MATLAB Function ==
  data: PRESSURE_H input; pressure output; PRESSURE_L input; PRESSURE_XL input
function pressure = fcn(PRESSURE_H, PRESSURE_L, PRESSURE_XL)

pressure = LPS25_convertPressure(PRESSURE_H, PRESSURE_L, PRESSURE_XL);

== matlab function FC_Test/Sensor Board/ICM42688/Configure/RunConfig/ConfigureSensors/SetFilters/Set Gyro AAF/MATLAB Function ==
  data: dataRead input; val output
function val = setGyroStatic2(dataRead)

val = bitor(dataRead, 0x03);

== matlab function FC_Test/Sensor Board/ICM42688/Configure/RunConfig/ConfigureSensors/SetFilters/Set Gyro AAF/MATLAB Function1 ==
  data: dataRead input; val output; delta input
function val = setGyroStatic2(dataRead, delta)

    % Clear bits 1:6 (equivalent to dataRead &= ~(0x3F);)
    dataRead = bitand(dataRead, uint8(~0x3F));
    
    % Set bits using sensors.ICM42688.config.gyro.AAF.DELT (equivalent to dataRead |= sensors.ICM42688.config.gyro.AAF.DELT;)
    dataRead = bitor(dataRead, delta);
    
    % Optionally, if you need to perform the operation below, you can uncomment this:
    % val = bitor(dataRead, 0x03); 
    
    % Assign the result to val
    val = dataRead;
    
end

== matlab function FC_Test/Sensor Board/ICM42688/Configure/RunConfig/ConfigureSensors/SetFilters/Set Accel AAF/MATLAB Function ==
  data: dataRead input uint8; val output uint8; delta input
function val = getAAF_Delta(dataRead, delta)

% Clear bits 1:6 (equivalent to dataRead &= ~(0x3F);)
dataRead = bitand(dataRead, uint8(~0x3F));

dataRead = bitor(dataRead, bitshift(delta, 0x01));

% Set the least significant bit (equivalent to dataRead |= 0x01;)
dataRead = bitor(dataRead, 1);

% Assign the result to val
val = dataRead;
